simulink model "PMSMDrive"  (R2023b)
settings: Solver=FixedStepDiscrete  StartTime=0.0  StopTime=2  RelTol=1e-3  EnableMultiTasking=on
PreLoadFcn:
  | Ts=2e-6;
libraries: spsThreePhaseSourceLib x1, electricdrivelib x1, spsStairGeneratorLib x1, spspowerguiLib x1
settings Model: Creator=The MathWorks, Inc.  LastModifiedBy=peter
settings SolverCC: AlgebraicLoopSolver=TrustRegion
settings DataIOCC: LimitDataPoints=on  SaveFormat=Array  SaveOutput=off  SignalLogging=off  SaveTime=off  ReturnWorkspaceOutputs=off  SignalLoggingName=sigsOut
settings OptimizationCC: ExpressionDepthLimit=2147483647  InitFltsAndDblsToZero=on  LifeSpan=inf
settings DebuggingCC: UnderspecifiedInitializationDetection=Classic  MergeDetectMultiDrivingBlocksExec=none  CheckExecutionContextPreStartOutputMsg=on  SignalResolutionControl=TryResolveAllWithWarning  MultiTaskDSMMsg=warning  MultiTaskCondExecSysMsg=none  FcnCallInpInsideContextMsg=warning  UnconnectedInputMsg=warning  UnconnectedOutputMsg=warning  UnconnectedLineMsg=warning  StateNameClashWarn=warning  SFUnexpectedBacktrackingDiag=warning  SFNoUnconditionalDefaultTransitionDiag=warning  SFExecutionAtInitializationDiag=none  ArithmeticOperatorsInVariantConditions=warning
settings HardwareCC: ProdBitPerPointer=32  ProdBitPerSizeT=32  ProdBitPerPtrDiffT=32  ProdLargestAtomicFloat=None  ProdIntDivRoundTo=Undefined  ProdEndianess=Unspecified  ProdWordSize=32  ProdHWDeviceType=32-bit Generic  TargetUnknown=on
settings ModelReferenceCC: EnableRefExpFcnMdlSchedulingChecks=on  PropagateSignalLabelsOutOfModel=off
settings SFSimCC: SimUseLocalCustomCode=off  CustomCodeUndefinedFunction=UseInterfaceOnly
settings RTWCC: RTWUseLocalCustomCode=off
settings CodeAppCC: StateflowObjectComments=on
settings GRTTargetCC: TargetLangStandard=C89/C90 (ANSI)  CombineOutputUpdateFcns=off  GRTInterface=on
settings ConfigComp: CovMetricSettings=dw  CovSaveCumulativeToWorkspaceVar=on  CovSaveSingleToWorkspaceVar=on  CovExternalEMLEnable=off  CovSFcnEnable=off
settings SimscapeCC: SimscapeNormalizeSystem=off

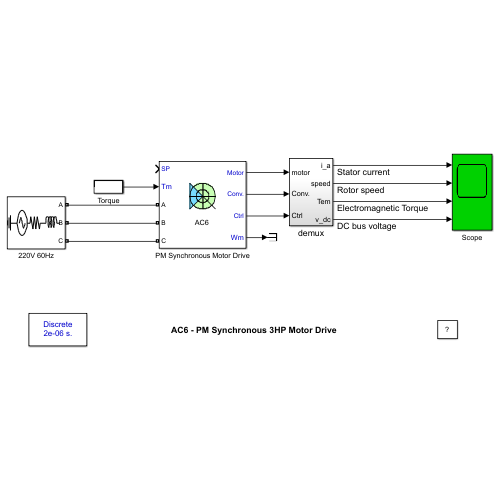
[thumbnail: Simulink's stored preview of the top-level diagram]
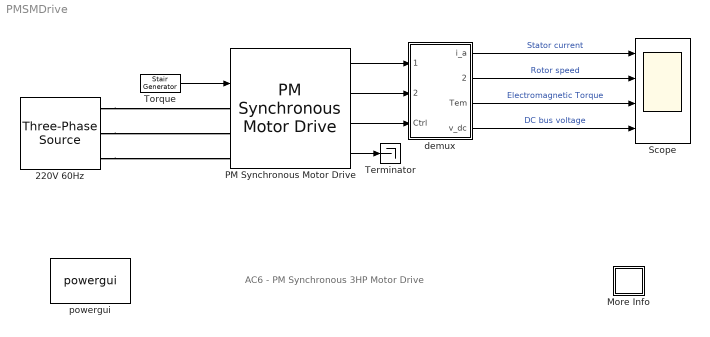
== system PMSMDrive ==
  note: AC6 - PM Synchronous 3HP Motor Drive
  220V 60Hz : spsThreePhaseSourceLib/Three-Phase Source  InternalConnection=Yg  VoltagePhases=off  Voltage=220  PhaseAngle=0  Voltage_phases=[25e3 25e3 25e3]/sqrt(3)  PhaseAngles_phases=[0 -120 +120]  Frequency=60  NonIdealSource=on  SpecifyImpedance=off  Resistance=0.02  Inductance=0.05e-3  ShortCircuitLevel=100e6  BaseVoltage=25e3  XRratio=7  BusType=swing  Pref=0  Qref=0  Prefabc=[10e3, 10e3, 10e3]  Qrefabc=[0, 0, 0]  Qmin=-inf  Qmax=inf
  More Info : Subsystem
      settings: OpenFcn="showExample(\"simscapeelectricalsps/PMSMDriveExample\")"
      mask Display: disp('?')
  PM Synchronous Motor Drive : electricdrivelib/AC drives/PM Synchronous Motor Drive  Rs=0.2  Lls=8.5e-3  Lms=8.5e-3  MachineConstant=Flux linkage established by magnets (V.s)  FluxCst=0.175  VoltageCst=126.966  TorqueCst=1.05  ia=0  ib=0  J=0.089  Friction=0.005  p=4  wm=0  thetam=0  Rsnb_rec=10e3  Csnb_rec=20e-9  Ron_rec=1e-3  Vf_rec=1.3  cap_bus=2000e-6  Rbrake=8  fbrake=4000  activationVoltage=320  shutdownVoltage=310  sourceFrequency=60  deviceType=IGBT / Diodes  Ron_inv=1e-3  Vf_inv=0.8  Vfd_inv=0.8  Tf=1e-6  Tt=2e-6  Tf_GTO=0  Tt_GTO=0  Rsnb_inv=5000  Csnb_inv=inf  regulationType=Speed regulation  Acc=1000  Dec=-1000  kp_sc=5  ki_sc=100  fc_sc=100  Tsc=7*20e-6  Tmin=-17.8  Tmax=17.8  modulationType=Hysteresis  h=0.1  kp_Id=200  ki_Id=1000  kp_Iq=200  ki_Iq=1000  fc_bus=50  car_freq=20000  freq_max=20e3  Tvect=20e-6  zeta=0.9  Trd=0.1  bwRatio=30  baseSampleTime=2e-06  outputBusMode=Multiple output buses  busLabels=off  MechanicalLoad=Torque Tm  modelDetailLevel=Detailed  driveType=AC6  AverageValue=off
  Scope : Scope  NumInputPorts=4
  Terminator : Terminator
  Torque : spsStairGeneratorLib/Stair Generator  t=[0.5 1.5]  e=[11 -11]  Ts=Ts
  demux : Subsystem
  powergui : spspowerguiLib/powergui  Priority=2  SimulationMode=Discrete  SampleTime=Ts  frequency=60  Iterations=50  frequencyindice=60  Pbase=100e6  ErrMax=1e-4  UnitsV=kV  UnitsW=MW  buscounter=0  FunctionMessages=off  echomessages=off  EnableUseOfTLC=off  CurrentSourceSwitches=off  DisableSnubberDevices=off  DisableRonSwitches=off  DisableVfSwitches=off  DisplayEquations=off  AutomaticDiscreteSolvers=off  SolverType=Tustin/Backward Euler (TBE)  Interpol=off  ExternalGateDelay=off  methode=off  Ts=0  x0status=blocks  SPID=off  SwTol=0  HookPort=off  NonlinearTolerance=1e-4  nMaxIteration=100  ContinueOnMaxIteration=off  RestoreLinks=warning  ResistiveCurrentMeasurement=off  Frange=[0:2:500]  Ylog=off  Xlog=on  ShowGrid=off  save=off  variable=ZData  structure=0  ZoomFFT=on  StartTime=0.0  cycles=1  DisplayStyle=1  fundamental=60  FreqAxis=off  MaxFrequency=1000  frequencyindicesteady=1  RmsSteady=1  display=off
  wires:
  Torque/1 -> PM Synchronous Motor Drive/2
  PM Synchronous Motor Drive/1 -> demux/1(motor)
  PM Synchronous Motor Drive/2 -> demux/2(Conv.)
  PM Synchronous Motor Drive/3 -> demux/3(Ctrl)
  demux/1(i_a) -> Scope/1  "Stator current"
  demux/2(speed) -> Scope/2  "Rotor speed"
  demux/3(Tem) -> Scope/3  "Electromagnetic Torque"
  demux/4(v_dc) -> Scope/4  "DC bus voltage"
  PM Synchronous Motor Drive/4 -> Terminator/1
  connections:
  220V 60Hz/RConn1 -- PM Synchronous Motor Drive/LConn1
  220V 60Hz/RConn2 -- PM Synchronous Motor Drive/LConn2
  220V 60Hz/RConn3 -- PM Synchronous Motor Drive/LConn3

== system PMSMDrive/More Info ==

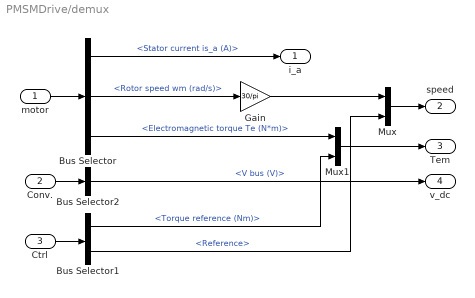
== system PMSMDrive/demux ==
  motor : Inport
  Conv. : Inport  Port=2
  Ctrl : Inport  Port=3
  Bus Selector : BusSelector  OutputSignals=Stator current is_a (A),Rotor speed wm (rad/s),Electromagnetic torque Te (N*m)
  Bus Selector1 : BusSelector  OutputSignals=Torque reference (Nm),Reference
  Bus Selector2 : BusSelector  OutputSignals=V bus (V)
  Gain : Gain  Gain=30/pi  SaturateOnIntegerOverflow=on  OutDataTypeStr=Inherit: Same as input  ParamDataTypeStr=Inherit: Same as input
  Mux : Mux  Inputs=2
  Mux1 : Mux  Inputs=2
  i_a : Outport  VectorParamsAs1DForOutWhenUnconnected=off
  speed : Outport  Port=2  VectorParamsAs1DForOutWhenUnconnected=off
  Tem : Outport  Port=3  VectorParamsAs1DForOutWhenUnconnected=off
  v_dc : Outport  Port=4  VectorParamsAs1DForOutWhenUnconnected=off
  wires:
  Bus Selector/2 -> Gain/1  "<Rotor speed wm (rad/s)>"
  Bus Selector2/1 -> v_dc/1  "<V bus (V)>"
  Conv./1 -> Bus Selector2/1
  Ctrl/1 -> Bus Selector1/1
  Bus Selector1/1 -> Mux1/2  "<Torque reference (Nm)>"
  Bus Selector1/2 -> Mux/2  "<Reference>"
  Gain/1 -> Mux/1
  Bus Selector/1 -> i_a/1  "<Stator current is_a (A)>"
  Bus Selector/3 -> Mux1/1  "<Electromagnetic torque Te (N*m)>"
  Mux1/1 -> Tem/1
  Mux/1 -> speed/1
  motor/1 -> Bus Selector/1
